simulink model "Microgrid_transition_model_111821_ben"  (R2020a)
settings: Solver=VariableStepAuto  StartTime=0.0  StopTime=16  MaxStep=1e-4  RelTol=1e-3
PreLoadFcn:
  | %run('FC_microgrid_param.m')
  | %load('gen_grid_init.mat')
InitFcn:
  | %load myisoModel_init;
  | run('FC_microgrid_param.m')
  | tic
  | run('CARTinitFcn.m')
  | %caseNo = 2;
  | 
  | %if (caseNo == 1)
  | %set_param(['Isolated_grid_paper_model_022521/SignalGen'], 'ActiveScenario', 'PStep222kW');
  | %else
  | %set_param(['Isolated_grid_paper_model_022521/SignalGen'], 'ActiveScenario', 'QStep222kVAr');
  | 
  | %end;
StopFcn:
  | toc
undefined symbols (not defined in the file): breakpoints1, breakpoints2, cc_kp, cp_table_data, ctrl, D1, Delta, DiscIntNeverNeededParam, DT, FC_BESS, FC_PV_FirstSolar, find_system, gcbh, libFC_BESS, libFC_PV, LowerLimit, magnitude, oversize, pll_ki, pll_kp, pq_ts, sps_rtmsupport, timer, Ts, ts, Ts_APC, Ts_Control, Ts_Power, UpperLimit
libraries: powerlib x152, powerlib_extras x100, simulink x95, powerlib_meascontrol x86, eePowerMeasurement x26, pi_ctrl x16, simulink_extras x12, sps_avr x7, spsDieselMotorModel x3, libFSArray x2, SignalEditorBlockLib x2, libLgBattery x1
(part 9 of 14)

== system Microgrid_transition_model_111821_ben/Wind Turbine Type 4/Control/Grid-Side Inverter Control/PI with anti-windup and dynamic limits - Iq ==
  note: Aramis Schwanka Trevisan - 16.08.2016
      | PI-controller with anti-windup and dynamic limits
      | Update 17.12.2016: External reset
      | Update 21.02.2017: External reset + limitation
  UpperLimit : Inport
  Input : Inport  Port=2
  LowerLimit : Inport  Port=3
  Reset : Inport  Port=4
  x_reset : Inport  Port=5
  Add1 : Sum
  Add2 : Sum
  Add3 : Sum  Inputs=+++
  Compare To Zero : simulink/Logic and Bit Operations/Compare To Zero  relop=>  OutDataTypeStr=uint8  ZeroCross=off
  Compare To Zero1 : simulink/Logic and Bit Operations/Compare To Zero  relop=<  OutDataTypeStr=uint8  ZeroCross=off
  Constant : Constant  Value=0
  Discrete Integrator : DiscreteIntegrator  IntegratorMethod=Integration: Trapezoidal  gainval=1  ExternalReset=sampled level  InitialConditionSource=external  InitialCondition=Init  SampleTime=Ts  UpperSaturationLimit=UpperLimit  LowerSaturationLimit=LowerLimit  ShowStatePort=on  ICPrevOutput=DiscIntNeverNeededParam  ICPrevScaledInput=DiscIntNeverNeededParam
  IC : InitialCondition  Value=Init
  Kp1 : Gain  Gain=Kp  SaturateOnIntegerOverflow=on  SampleTime=Ts  OutDataTypeStr=Inherit: Same as input  ParamDataTypeStr=Inherit: Same as input
  Kp5 : Gain  Gain=Ki  SaturateOnIntegerOverflow=on  SampleTime=Ts  OutDataTypeStr=Inherit: Same as input  ParamDataTypeStr=Inherit: Same as input
  Logical Operator : Logic  AllPortsSameDT=off  OutDataTypeStr=boolean
  Logical Operator1 : Logic  AllPortsSameDT=off  OutDataTypeStr=boolean
  Logical Operator2 : Logic  Operator=OR  AllPortsSameDT=off  OutDataTypeStr=boolean
  Logical Operator3 : Logic  Operator=OR  Inputs=3  AllPortsSameDT=off  OutDataTypeStr=boolean
  Logical Operator4 : Logic  Operator=NOT  Inputs=3  AllPortsSameDT=off  OutDataTypeStr=boolean
  Product : Product  Inputs=3
  Product1 : Product  Inputs=3
  Product2 : Product
  Relational Operator : RelationalOperator  OutDataTypeStr=boolean  RndMeth=Nearest
  Relational Operator1 : RelationalOperator  Operator=<=  OutDataTypeStr=boolean  RndMeth=Nearest
  Relational Operator2 : RelationalOperator  OutDataTypeStr=boolean  RndMeth=Nearest
  Relational Operator3 : RelationalOperator  Operator=<=  OutDataTypeStr=boolean  RndMeth=Nearest
  Saturation Dynamic : simulink/Discontinuities/Saturation Dynamic  OutMin=[]  OutMax=[]  OutDataTypeStr=Inherit: Same as second input  OutDataType=fixdt(1, 16)  OutScaling=2^-10  DoSatur=off
  Switch : Switch  Criteria=u2 > Threshold
  Zero-Order Hold : ZeroOrderHold  SampleTime=Ts
  Output : Outport
  wires:
  Saturation Dynamic/1 -> Output/1
  Reset/1 -> Product2/2, Logical Operator3/3, Logical Operator4/1
  IC/1 -> Discrete Integrator/3
  Switch/1 -> Discrete Integrator/1
  Compare To Zero1/1 -> Logical Operator1/2  "Error_is_negative"
  Logical Operator/1 -> Logical Operator2/1
  Relational Operator/1 -> Logical Operator/1  "UpperLimit_is_Reached"
  Relational Operator1/1 -> Logical Operator1/1  "LowerLimit_Is_Reached"
  Logical Operator2/1 -> Switch/2
  Kp1/1 -> Zero-Order Hold/1
  Constant/1 -> Switch/1
  Kp5/1 -> Switch/3
  Add2/1 -> Saturation Dynamic/2
  Zero-Order Hold/1 -> Add2/1, Add1/2
  Add1/1 -> Relational Operator/1, Relational Operator1/1
  Input/1 -> Kp5/1, Compare To Zero1/1, Compare To Zero/1, Kp1/1
  Compare To Zero/1 -> Logical Operator/2  "Error_is_positive"
  Logical Operator1/1 -> Logical Operator2/2
  Relational Operator2/1 -> Logical Operator3/1, Product/2
  Relational Operator3/1 -> Product1/2, Logical Operator3/2
  Logical Operator3/1 -> Discrete Integrator/2
  Add3/1 -> IC/1
  Product1/1 -> Add3/2
  UpperLimit/1 -> Saturation Dynamic/1, Relational Operator/2, Product/1, Relational Operator2/2
  Discrete Integrator/State -> Add1/1, Relational Operator3/1, Relational Operator2/1
  Discrete Integrator/1 -> Add2/2
  Logical Operator4/1 -> Product/3, Product1/1
  LowerLimit/1 -> Saturation Dynamic/3, Relational Operator1/2, Relational Operator3/2, Product1/3
  Product2/1 -> Add3/3
  Product/1 -> Add3/1
  x_reset/1 -> Product2/1

== system Microgrid_transition_model_111821_ben/Wind Turbine Type 4/Control/Grid-Side Inverter Control/Predictor1 ==
  in : Inport
  Delay : Delay  DelayLength=1  InitialCondition=Init_value  SampleTime=Ts
  Delay1 : Delay  DelayLength=1  InitialCondition=Init_value  SampleTime=Ts
  Gain : Gain  Gain=2
  Sum1 : Sum  Inputs=|+-
  out : Outport
  wires:
  in/1 -> Delay/1
  Delay1/1 -> Sum1/2
  Sum1/1 -> out/1
  Delay/1 -> Gain/1, Delay1/1
  Gain/1 -> Sum1/1

== system Microgrid_transition_model_111821_ben/Wind Turbine Type 4/Control/Grid-Side Inverter Control/Predictor2 ==
  in : Inport
  Delay : Delay  DelayLength=1  InitialCondition=Init_value  SampleTime=Ts
  Delay1 : Delay  DelayLength=1  InitialCondition=Init_value  SampleTime=Ts
  Gain : Gain  Gain=2
  Sum1 : Sum  Inputs=|+-
  out : Outport
  wires:
  Gain/1 -> Sum1/1
  Delay/1 -> Delay1/1, Gain/1
  Sum1/1 -> out/1
  Delay1/1 -> Sum1/2
  in/1 -> Delay/1

== system Microgrid_transition_model_111821_ben/Wind Turbine Type 4/Control/Measurement and Transformation/Discrete 3-phase PLL-Driven Positive-Sequence Active & Reactive Power ==
  note: Pierre Giroux, Gilbert Sybille
      | Power System Simulation Laboratory
      | IREQ, Hydro-Quebc
  note: Discrete 3-phase PLL-driven Positive-Sequence Active & Reactive Power
  Freq : Inport  PortDimensions=1
  w : Inport  Port=2  PortDimensions=1
  Vabc : Inport  Port=3  PortDimensions=3
  Iabc : Inport  Port=4  PortDimensions=3
  Deg->Rad : Gain  Gain=pi/180  SaturateOnIntegerOverflow=on  OutDataTypeStr=Inherit: Same as input  ParamDataTypeStr=Inherit: Same as input
  Discrete 3-phase PLL-Driven Positive-Sequence Fundamental Value : Subsystem  mask(Discrete 3-phase PLL-Driven Positive-Sequence Fundamental Value){Finit=Finit, Fmin=Fmin, Par_Init=Par_Vinit, Ts=Ts}
      mask prompts: Finit "Initial frequency (Hz):"; Fmin "Minimum frequency (Hz):"; Par_Init "Initial input (positive component): [ Mag  Phase-relative-to-PLL(degrees) ]"; Ts "Sample time:"
      mask help:
      | For a supplied fundamental frequency (port Freq), this discrete block computes  the positive-sequence component (Magnitude and Phase)  of a set of three balanced or unbalanced signals (port abc) which may contain harmonics.
      |  Input port "Sin_Cos" (a two-dimension signal) provides the reference frame required for the computation..
      |  First and second outputs return respectively the magnitude and phase (in degrees relative to the PLL phase)) of the fundamental.
      | For the first cycle of simulation, the outputs are held constant to the values specified by the parameter "Initial input".
      | constant to the values specified by the parameter "Initial input". The value of the parameter "Minimum frequency" is used to determine the buffer size of the "Variable Transport Delay" block found inside this subsystem.
      mask init:
      | Real_Init=Par_Init(1)*cos(pi/180*Par_Init(2));
      | Imag_Init=Par_Init(1)*sin(pi/180*Par_Init(2));
      | power_initmask();
      settings: OpenFcn=power_openblockproxy();
  Discrete 3-phase PLL-Driven Positive-Sequence Fundamental Value2 : Subsystem  mask(Discrete 3-phase PLL-Driven Positive-Sequence Fundamental Value){Finit=Finit, Fmin=Fmin, Par_Init=Par_Iinit, Ts=Ts}
      mask prompts: Finit "Initial frequency (Hz):"; Fmin "Minimum frequency (Hz):"; Par_Init "Initial input (positive component): [ Mag  Phase-relative-to-PLL(degrees) ]"; Ts "Sample time:"
      mask help:
      | For a supplied fundamental frequency (port Freq), this discrete block computes  the positive-sequence component (Magnitude and Phase)  of a set of three balanced or unbalanced signals (port abc) which may contain harmonics.
      |  Input port "Sin_Cos" (a two-dimension signal) provides the reference frame required for the computation..
      |  First and second outputs return respectively the magnitude and phase (in degrees relative to the PLL phase)) of the fundamental.
      | For the first cycle of simulation, the outputs are held constant to the values specified by the parameter "Initial input".
      | constant to the values specified by the parameter "Initial input". The value of the parameter "Minimum frequency" is used to determine the buffer size of the "Variable Transport Delay" block found inside this subsystem.
      mask init:
      | Real_Init=Par_Init(1)*cos(pi/180*Par_Init(2));
      | Imag_Init=Par_Init(1)*sin(pi/180*Par_Init(2));
      | power_initmask();
      settings: OpenFcn=power_openblockproxy();
  Gain1 : Gain  Gain=3/2  SaturateOnIntegerOverflow=on  OutDataTypeStr=Inherit: Same as input  ParamDataTypeStr=Inherit: Same as input
  Mux2 : Mux  Inputs=2
  Mux3 : Mux  Inputs=2
  Product : Product  InputSameDT=on  SaturateOnIntegerOverflow=on  OutDataTypeStr=Inherit: Same as first input
  Product1 : Product  InputSameDT=on  SaturateOnIntegerOverflow=on  OutDataTypeStr=Inherit: Same as first input
  Product2 : Product  InputSameDT=on  SaturateOnIntegerOverflow=on  OutDataTypeStr=Inherit: Same as first input
  Sum : Sum  Inputs=+-  InputSameDT=on  SaturateOnIntegerOverflow=on  OutDataTypeStr=Inherit: Same as first input
  Trigonometric Function : Trigonometry
  Trigonometric Function1 : Trigonometry  Operator=cos
  Mag_V_I : Outport  VectorParamsAs1DForOutWhenUnconnected=off
  P_Q : Outport  Port=2  VectorParamsAs1DForOutWhenUnconnected=off
  wires:
  Iabc/1 -> Discrete 3-phase PLL-Driven Positive-Sequence Fundamental Value2/3(abc)
  Discrete 3-phase PLL-Driven Positive-Sequence Fundamental Value2/1(Mag) -> Product2/2, Mux3/2
  Product2/1 -> Product1/2, Product/1
  Gain1/1 -> P_Q/1
  Mux3/1 -> Mag_V_I/1
  Product1/1 -> Mux2/2
  Product/1 -> Mux2/1
  Mux2/1 -> Gain1/1
  Trigonometric Function/1 -> Product1/1
  Trigonometric Function1/1 -> Product/2
  Deg->Rad/1 -> Trigonometric Function/1, Trigonometric Function1/1
  Sum/1 -> Deg->Rad/1
  Discrete 3-phase PLL-Driven Positive-Sequence Fundamental Value2/2(Phase) -> Sum/2
  Discrete 3-phase PLL-Driven Positive-Sequence Fundamental Value/1(Mag) -> Product2/1, Mux3/1
  Discrete 3-phase PLL-Driven Positive-Sequence Fundamental Value/2(Phase) -> Sum/1
  w/1 -> Discrete 3-phase PLL-Driven Positive-Sequence Fundamental Value2/2(w), Discrete 3-phase PLL-Driven Positive-Sequence Fundamental Value/2(w)
  Freq/1 -> Discrete 3-phase PLL-Driven Positive-Sequence Fundamental Value2/1(Freq), Discrete 3-phase PLL-Driven Positive-Sequence Fundamental Value/1(Freq)
  Vabc/1 -> Discrete 3-phase PLL-Driven Positive-Sequence Fundamental Value/3(abc)

== system Microgrid_transition_model_111821_ben/Wind Turbine Type 4/Control/Measurement and Transformation/Extract References ==
  v_abc : Inport
  Extract References : Subsystem
  Mux : Mux  Inputs=3
  Voltage and Frequency Protection : Subsystem
  rad/s to Hz : Gain  Gain=1/2/pi
  u_frt_pu : Outport
  protection_u_f : Outport  Port=2
  references : Outport  Port=3
  wires:
  Extract References/4(u_frt_pu) -> u_frt_pu/1
  Extract References/2(wt_ref) -> Mux/2
  Extract References/3(w_ref) -> rad/s to Hz/1, Mux/3
  Mux/1 -> references/1
  [Vpos] -> Voltage and Frequency Protection/1(Vpos)
  [fgrid] -> Voltage and Frequency Protection/2(fgrid)
  Voltage and Frequency Protection/1(u_f_protect) -> protection_u_f/1
  Extract References/1(u_ref) -> [Vpos], Mux/1
  rad/s to Hz/1 -> [fgrid]
  v_abc/1 -> Extract References/1(v_abc)

== system Microgrid_transition_model_111821_ben/Wind Turbine Type 4/Control/Measurement and Transformation/Filter ==
  Vabc_grid : Inport
  Iabc_grid_conv : Inport  Port=2
  Vabc_LL_s : Inport  Port=3
  Iabc_stator : Inport  Port=4
  IL : Inport  Port=5
  Vdc : Inport  Port=6
  Qref : Inport  Port=7
  wr : Inport  Port=8
  angle_rotor : Inport  Port=9
  Second-Order Filter{,1..6} (7 alike) : powerlib_meascontrol/Filters/Second-Order Filter  FilterType=Lowpass  Fo=Freq  Zeta=Zeta  Ts=Ts  Initialize=off  Vac_Init="[0,  0,  60]"  Vdc_Init=0  PlotResponse=off  FreqRange=[0, 500, 1]
      settings: SourceProductBaseCode=MT,PS
  Second-Order Filter7 : powerlib_meascontrol/Filters/Second-Order Filter  FilterType=Lowpass  Fo=Freq  Zeta=Zeta  Ts=Ts  Initialize=on  Vac_Init=[0.8 -25 60]*0  Vdc_Init=Vdc_nom  PlotResponse=off  FreqRange=[0, 500, 1]
      settings: SourceProductBaseCode=MT,PS
  Second-Order Filter8 : powerlib_meascontrol/Filters/Second-Order Filter  FilterType=Lowpass  Fo=Freq  Zeta=Zeta  Ts=Ts  Initialize=on  Vac_Init=[0.8 -25 60]*0  Vdc_Init=1+init(1)/100  PlotResponse=off  FreqRange=[0, 500, 1]
      settings: SourceProductBaseCode=MT,PS
  "Vabc_grid " : Outport  VectorParamsAs1DForOutWhenUnconnected=off
  "Iabc_grid_conv " : Outport  Port=2  VectorParamsAs1DForOutWhenUnconnected=off
  "Vabc_LL_s " : Outport  Port=3  VectorParamsAs1DForOutWhenUnconnected=off
  "Iabc_stator " : Outport  Port=4  VectorParamsAs1DForOutWhenUnconnected=off
  "IL " : Outport  Port=5  VectorParamsAs1DForOutWhenUnconnected=off
  "Vdc " : Outport  Port=6  VectorParamsAs1DForOutWhenUnconnected=off
  "Qref " : Outport  Port=7  VectorParamsAs1DForOutWhenUnconnected=off
  "wr " : Outport  Port=8  VectorParamsAs1DForOutWhenUnconnected=off
  "angle_rotor " : Outport  Port=9  VectorParamsAs1DForOutWhenUnconnected=off
  wires:
  angle_rotor/1 -> Second-Order Filter6/1
  Second-Order Filter6/1 -> "angle_rotor "/1
  Second-Order Filter/1 -> "Vabc_grid "/1
  Second-Order Filter1/1 -> "Iabc_grid_conv "/1
  Vdc/1 -> Second-Order Filter7/1
  Second-Order Filter7/1 -> "Vdc "/1
  Second-Order Filter3/1 -> "Iabc_stator "/1
  wr/1 -> Second-Order Filter8/1
  Second-Order Filter8/1 -> "wr "/1
  Qref/1 -> Second-Order Filter5/1
  Second-Order Filter5/1 -> "Qref "/1
  IL/1 -> Second-Order Filter4/1
  Second-Order Filter4/1 -> "IL "/1
  Vabc_grid/1 -> Second-Order Filter/1
  Iabc_grid_conv/1 -> Second-Order Filter1/1
  Vabc_LL_s/1 -> Second-Order Filter2/1
  Second-Order Filter2/1 -> "Vabc_LL_s "/1
  Iabc_stator/1 -> Second-Order Filter3/1

== system Microgrid_transition_model_111821_ben/Wind Turbine Type 4/Control/Measurement and Transformation/Stator flux estimator ==
  note: Quasi steady state flux at generator stator
  Vdqs : Inport
  Idqs : Inport  Port=2
  wr : Inport  Port=3
  Divide2 : Product  Inputs=**
  Divide4 : Product  Inputs=*/
  Divide7 : Product  Inputs=**
  Divide8 : Product  Inputs=*/
  First-Order Filter : powerlib_meascontrol/Filters/First-Order Filter  FilterType=Lowpass  Tc=Flux_meas_time_constant  Ts=Ts  Initialize=on  Vac_Init=[0, 0, 0]  Vdc_Init=1  PlotResponse=off  FreqRange="[0,  200,  1]"
      settings: SourceProductBaseCode=MT,PS
  Gain : Gain  Gain=-1
  Magnitude of flux : Fcn  Expr=sqrt(u(1)^2+u(2)^2)
  Mux1 : Mux  Inputs=2
  Rs2 : Constant  Value=Resistance
  Rs4 : Constant  Value=Resistance
  Selector1 : Selector  InputPortWidth=2  IndexOptions=Index vector (dialog)  Indices=2  OutputSizes=1
  Selector3 : Selector  InputPortWidth=2  IndexOptions=Index vector (dialog)  Indices=2  OutputSizes=1
  Selector7 : Selector  InputPortWidth=2  IndexOptions=Index vector (dialog)  Indices=1  OutputSizes=1
  Selector8 : Selector  InputPortWidth=2  IndexOptions=Index vector (dialog)  Indices=1  OutputSizes=1
  Sum2 : Sum  Inputs=|+-
  Sum4 : Sum  Inputs=|+-
  avoid division by 0 : Saturate  UpperLimit=inf  LowerLimit=1e-6
  Flux : Outport  VectorParamsAs1DForOutWhenUnconnected=off
  wires:
  First-Order Filter/1 -> Flux/1
  avoid division by 0/1 -> Gain/1, Divide4/2
  Magnitude of flux/1 -> First-Order Filter/1
  Mux1/1 -> Magnitude of flux/1
  Divide8/1 -> Mux1/2  "phi_q"
  Gain/1 -> Divide8/2
  Sum4/1 -> Divide8/1
  Selector8/1 -> Divide7/1  "Id"
  Rs4/1 -> Divide7/2
  Selector7/1 -> Sum4/1  "Vd"
  Divide7/1 -> Sum4/2  "Rs*Id"
  Idqs/1 -> Selector8/1, Selector3/1
  Vdqs/1 -> Selector7/1, Selector1/1
  Selector3/1 -> Divide2/1  "Iq"
  Rs2/1 -> Divide2/2
  Selector1/1 -> Sum2/1  "Vq"
  Divide2/1 -> Sum2/2  "Rs*Iq"
  Divide4/1 -> Mux1/1  "phi_d"
  Sum2/1 -> Divide4/1
  wr/1 -> avoid division by 0/1

== system Microgrid_transition_model_111821_ben/Wind Turbine Type 4/Control/Measurement and Transformation/abc2qd ==
  note: This subsystem converts Vab and Vbc to Vd,Vq. The sine and cosine com-
      | puted here are sent to the inverse transformation subsystem qd/abc.
  Vabc_LL : Inport
  sin_cos : Inport  Port=2
  Fcn2 : Fcn  Expr=(u[4]*(2*u[1]+u[2]) + (sqrt(3)*u[2]*u[3])) * 1/3
  Fcn3 : Fcn  Expr=(u[3]*(2*u[1]+u[2]) + (-sqrt(3)*u[2]*u[4])) * 1/3
  Mux : Mux  Inputs=2
  Mux1 : Mux  Inputs=[ 2 2 ]
  Selector : Selector  InputPortWidth=3  IndexOptions=Index vector (dialog)  Indices=[1 2]  OutputSizes=1
  Vdq : Outport  InitialOutput=0  VectorParamsAs1DForOutWhenUnconnected=off
  wires:
  Fcn3/1 -> Mux/1
  Fcn2/1 -> Mux/2
  Mux1/1 -> Fcn3/1, Fcn2/1
  Vabc_LL/1 -> Selector/1
  sin_cos/1 -> Mux1/2
  Mux/1 -> Vdq/1
  Selector/1 -> Mux1/1

== system Microgrid_transition_model_111821_ben/Wind Turbine Type 4/Control/Speed & Pitch Control1/Discrete PI Controller1 ==
  note: Discrete PID Controller
  note: Pierre Giroux, Gilbert Sybille
      | Power System Simulation Laboratory
      | IREQ, Hydro-Quebc
  Error : Inport  SampleTime=Ts
  Discrete-Time Integrator : DiscreteIntegrator  InitialCondition=Init  SampleTime=Ts  LimitOutput=on  UpperSaturationLimit=UpperLimit  LowerSaturationLimit=LowerLimit  ICPrevOutput=DiscIntNeverNeededParam  ICPrevScaledInput=DiscIntNeverNeededParam
  Kp4 : Gain  Gain=Kp  SaturateOnIntegerOverflow=on  SampleTime=Ts  OutDataTypeStr=Inherit: Same as input  ParamDataTypeStr=Inherit: Same as input
  Kp5 : Gain  Gain=Ki  SaturateOnIntegerOverflow=on  SampleTime=Ts  OutDataTypeStr=Inherit: Same as input  ParamDataTypeStr=Inherit: Same as input
  Saturation2 : Saturate  UpperLimit=UpperLimit  LowerLimit=LowerLimit  SampleTime=Ts
  Sum6 : Sum  InputSameDT=on  SaturateOnIntegerOverflow=on  SampleTime=Ts  OutDataTypeStr=Inherit: Same as first input
  Zero-Order Hold : ZeroOrderHold  SampleTime=Ts
  Out : Outport  SampleTime=Ts  InitialOutput=0  VectorParamsAs1DForOutWhenUnconnected=off
  wires:
  Zero-Order Hold/1 -> Sum6/1
  Saturation2/1 -> Out/1
  Discrete-Time Integrator/1 -> Sum6/2
  Kp4/1 -> Zero-Order Hold/1
  Kp5/1 -> Discrete-Time Integrator/1
  Sum6/1 -> Saturation2/1
  Error/1 -> Kp5/1, Kp4/1

== system Microgrid_transition_model_111821_ben/Wind Turbine Type 4/Control/Speed & Pitch Control1/Discrete PI Controller2 ==
  note: Discrete PID Controller
  note: Pierre Giroux, Gilbert Sybille
      | Power System Simulation Laboratory
      | IREQ, Hydro-Quebc
  Error : Inport  SampleTime=Ts
  Discrete-Time Integrator : DiscreteIntegrator  InitialCondition=Init  SampleTime=Ts  LimitOutput=on  UpperSaturationLimit=UpperLimit  LowerSaturationLimit=LowerLimit  ICPrevOutput=DiscIntNeverNeededParam  ICPrevScaledInput=DiscIntNeverNeededParam
  Kp4 : Gain  Gain=Kp  SaturateOnIntegerOverflow=on  SampleTime=Ts  OutDataTypeStr=Inherit: Same as input  ParamDataTypeStr=Inherit: Same as input
  Kp5 : Gain  Gain=Ki  SaturateOnIntegerOverflow=on  SampleTime=Ts  OutDataTypeStr=Inherit: Same as input  ParamDataTypeStr=Inherit: Same as input
  Saturation2 : Saturate  UpperLimit=UpperLimit  LowerLimit=LowerLimit  SampleTime=Ts
  Sum6 : Sum  InputSameDT=on  SaturateOnIntegerOverflow=on  SampleTime=Ts  OutDataTypeStr=Inherit: Same as first input
  Zero-Order Hold : ZeroOrderHold  SampleTime=Ts
  Out : Outport  SampleTime=Ts  InitialOutput=0  VectorParamsAs1DForOutWhenUnconnected=off
  wires:
  Zero-Order Hold/1 -> Sum6/1
  Saturation2/1 -> Out/1
  Discrete-Time Integrator/1 -> Sum6/2
  Kp4/1 -> Zero-Order Hold/1
  Kp5/1 -> Discrete-Time Integrator/1
  Sum6/1 -> Saturation2/1
  Error/1 -> Kp5/1, Kp4/1

== system Microgrid_transition_model_111821_ben/../Control/Grid-side converter Control system/INT/S6 ==
  note: Limiter
      | with external
      | limits
  MAX : Inport
  In : Inport  Port=2
  MIN : Inport  Port=3
  MinMax : MinMax  Function=max  Inputs=2  InputSameDT=on  SaturateOnIntegerOverflow=on
  MinMax1 : MinMax  Inputs=2  InputSameDT=on  SaturateOnIntegerOverflow=on
  "  " : Outport  InitialOutput=0  VectorParamsAs1DForOutWhenUnconnected=off
  wires:
  In/1 -> MinMax1/2
  MinMax/1 -> "  "/1
  MIN/1 -> MinMax/1
  MAX/1 -> MinMax1/1
  MinMax1/1 -> MinMax/2

== system Microgrid_transition_model_111821_ben/../Control/Measurement and Transformation/Discrete 3-phase PLL-Driven Positive-Sequence Active & Reactive Power/Discrete 3-phase PLL-Driven Positive-Sequence Fundamental Value ==
  note: Discrete 3-phase PLL-Driven Positive-Sequence Fundamental Value
  note: Pierre Giroux, Gilbert Sybille
      | Power System Simulation Laboratory
      | IREQ, Hydro-Quebc
  Freq : Inport
  w : Inport  Port=2  PortDimensions=1
  abc : Inport  Port=3  PortDimensions=3
  Cartesian to Polar : simulink_extras/Transformations/Cartesian to Polar
  Demux : Demux  Outputs=3
      settings: DisplayOption=none
  Discrete Variable Frequency Mean value1 : Subsystem  mask(Discrete Variable-Frequency Mean Value){Finit=Finit, Fmin=Fmin, Vinit=Imag_Init, Ts=Ts}
      mask prompts: Finit "Initial frequency (Hz):"; Fmin "Minimum frequency (Hz):"; Vinit "Initial input (DC component):"; Ts "Sample time:"
      mask help:
      | This discrete block computes the mean value of the input signal (port In) over a running window of one cycle of a specified frequency (port Freq).
      |
      | For the first cycle of simulation (specified by the parameter "Initial frequency"), the output is held to the value of the  "Initial input" parameter.
      |
      | The value of the parameter "Minimum frequency" is used to determine the buffer size of the "Variable Transport Delay" block found inside this subsystem.
      mask init:
      | MaxDelay=1/Fmin+Ts;
      | power_initmask();
      settings: OpenFcn=power_openblockproxy();
  Discrete Variable Frequency Mean value2 : Subsystem  mask(Discrete Variable-Frequency Mean Value){Finit=Finit, Fmin=Fmin, Vinit=Real_Init, Ts=Ts}
      mask prompts: Finit "Initial frequency (Hz):"; Fmin "Minimum frequency (Hz):"; Vinit "Initial input (DC component):"; Ts "Sample time:"
      mask help:
      | This discrete block computes the mean value of the input signal (port In) over a running window of one cycle of a specified frequency (port Freq).
      |
      | For the first cycle of simulation (specified by the parameter "Initial frequency"), the output is held to the value of the  "Initial input" parameter.
      |
      | The value of the parameter "Minimum frequency" is used to determine the buffer size of the "Variable Transport Delay" block found inside this subsystem.
      mask init:
      | MaxDelay=1/Fmin+Ts;
      | power_initmask();
      settings: OpenFcn=power_openblockproxy();
  Rad->Deg. : Gain  Gain=180/pi  SaturateOnIntegerOverflow=on  OutDataTypeStr=Inherit: Same as input  ParamDataTypeStr=Inherit: Same as input
  Terminator : Terminator
  abc to dq0 : powerlib_meascontrol/Transformations/abc to dq0  Alignment=90 degrees behind phase A axis
      settings: SourceProductBaseCode=MT,PS
  Mag : Outport  VectorParamsAs1DForOutWhenUnconnected=off
  Phase : Outport  Port=2  VectorParamsAs1DForOutWhenUnconnected=off
  wires:
  Cartesian to Polar/2 -> Rad->Deg./1
  Cartesian to Polar/1 -> Mag/1
  Demux/3 -> Terminator/1
  abc to dq0/1 -> Demux/1
  abc/1 -> abc to dq0/1
  Demux/1 -> Discrete Variable Frequency Mean value2/2(In)
  Demux/2 -> Discrete Variable Frequency Mean value1/2(In)
  Discrete Variable Frequency Mean value1/1(Mean) -> Cartesian to Polar/2  "Real"
  Rad->Deg./1 -> Phase/1
  Discrete Variable Frequency Mean value2/1(Mean) -> Cartesian to Polar/1  "Real"
  Freq/1 -> Discrete Variable Frequency Mean value1/1(Freq), Discrete Variable Frequency Mean value2/1(Freq)
  w/1 -> abc to dq0/2

== system Microgrid_transition_model_111821_ben/../Control/Measurement and Transformation/Discrete 3-phase PLL-Driven Positive-Sequence Active & Reactive Power/Discrete 3-phase PLL-Driven Positive-Sequence Fundamental Value2 ==
  note: Pierre Giroux, Gilbert Sybille
      | Power System Simulation Laboratory
      | IREQ, Hydro-Quebc
  note: Discrete 3-phase PLL-Driven Positive-Sequence Fundamental Value
  Freq : Inport
  w : Inport  Port=2  PortDimensions=1
  abc : Inport  Port=3  PortDimensions=3
  Cartesian to Polar : simulink_extras/Transformations/Cartesian to Polar
  Demux : Demux  Outputs=3
      settings: DisplayOption=none
  Discrete Variable Frequency Mean value1 : Subsystem  mask(Discrete Variable-Frequency Mean Value){Finit=Finit, Fmin=Fmin, Vinit=Imag_Init, Ts=Ts}
      mask prompts: Finit "Initial frequency (Hz):"; Fmin "Minimum frequency (Hz):"; Vinit "Initial input (DC component):"; Ts "Sample time:"
      mask help:
      | This discrete block computes the mean value of the input signal (port In) over a running window of one cycle of a specified frequency (port Freq).
      |
      | For the first cycle of simulation (specified by the parameter "Initial frequency"), the output is held to the value of the  "Initial input" parameter.
      |
      | The value of the parameter "Minimum frequency" is used to determine the buffer size of the "Variable Transport Delay" block found inside this subsystem.
      mask init:
      | MaxDelay=1/Fmin+Ts;
      | power_initmask();
      settings: OpenFcn=power_openblockproxy();
  Discrete Variable Frequency Mean value2 : Subsystem  mask(Discrete Variable-Frequency Mean Value){Finit=Finit, Fmin=Fmin, Vinit=Real_Init, Ts=Ts}
      mask prompts: Finit "Initial frequency (Hz):"; Fmin "Minimum frequency (Hz):"; Vinit "Initial input (DC component):"; Ts "Sample time:"
      mask help:
      | This discrete block computes the mean value of the input signal (port In) over a running window of one cycle of a specified frequency (port Freq).
      |
      | For the first cycle of simulation (specified by the parameter "Initial frequency"), the output is held to the value of the  "Initial input" parameter.
      |
      | The value of the parameter "Minimum frequency" is used to determine the buffer size of the "Variable Transport Delay" block found inside this subsystem.
      mask init:
      | MaxDelay=1/Fmin+Ts;
      | power_initmask();
      settings: OpenFcn=power_openblockproxy();
  Rad->Deg. : Gain  Gain=180/pi  SaturateOnIntegerOverflow=on  OutDataTypeStr=Inherit: Same as input  ParamDataTypeStr=Inherit: Same as input
  Terminator : Terminator
  abc to dq0 : powerlib_meascontrol/Transformations/abc to dq0  Alignment=90 degrees behind phase A axis
      settings: SourceProductBaseCode=MT,PS
  Mag : Outport  VectorParamsAs1DForOutWhenUnconnected=off
  Phase : Outport  Port=2  VectorParamsAs1DForOutWhenUnconnected=off
  wires:
  w/1 -> abc to dq0/2
  Freq/1 -> Discrete Variable Frequency Mean value2/1(Freq), Discrete Variable Frequency Mean value1/1(Freq)
  Discrete Variable Frequency Mean value2/1(Mean) -> Cartesian to Polar/1  "Real"
  Rad->Deg./1 -> Phase/1
  Discrete Variable Frequency Mean value1/1(Mean) -> Cartesian to Polar/2  "Real"
  Demux/2 -> Discrete Variable Frequency Mean value1/2(In)
  Demux/1 -> Discrete Variable Frequency Mean value2/2(In)
  abc/1 -> abc to dq0/1
  abc to dq0/1 -> Demux/1
  Demux/3 -> Terminator/1
  Cartesian to Polar/1 -> Mag/1
  Cartesian to Polar/2 -> Rad->Deg./1

== system Microgrid_transition_model_111821_ben/FC_BESS/SMAInverter/85_SMAControl/InvControl/40_V_Control ==
  Add1 : Sum  Inputs=+-
  Bus Creator : BusCreator  Inputs=1
  Bus Selector1 : BusSelector  OutputSignals=vdq0_inv  OutputAsBus=on
  Bus Selector8 : BusSelector  OutputSignals=use_csi,vdq
  Constant1 : Constant  Value=double(0)
  Constant2 : Constant  Value=10  OutDataTypeStr=double
  Demux : Demux  Outputs=2
  Demux1 : Demux  Outputs=2
  Logical Operator : Logic  Operator=NOT  Inputs=1  AllPortsSameDT=off  OutDataTypeStr=boolean
  Manual Switch2 : ManualSwitch  CurrentSetting=0
  Mux2 : Mux  Inputs=2
  Mux8 : Mux  Inputs=2
  PI_controller_with_reset : pi_ctrl/PI_controller_with_reset  Kp=0.0005  Ti=0.02  Ts=Ts  Iup=1.5  Idown=0  PIup=1.5  PIdown=0
  PI_controller_with_reset1 : pi_ctrl/PI_controller_with_reset  Kp=0.0005  Ti=0.02  Ts=Ts  Iup=1.5  Idown=-1  PIup=1.5  PIdown=-1
  Scope : Scope  NumInputPorts=4
  Selector : Selector  InputPortWidth=4  IndexOptions=Index vector (dialog)  Indices=2  OutputSizes=1
  Selector2 : Selector  InputPortWidth=3  IndexOptions=Index vector (dialog)  Indices=[1 2]  OutputSizes=1
  Subsystem : Subsystem  mask{Ts=Ts}
      mask prompts: Ts "Sampling time"
  Unit Delay : UnitDelay  SampleTime=-1  HasFrameUpgradeWarning=on
  Unit Delay1 : UnitDelay  InitialCondition=[0 0]  SampleTime=-1  HasFrameUpgradeWarning=on
  tag scope: V_Ctrl=scoped
  wires:
  Unit Delay1/1 -> Demux/1, Subsystem/3(init)
  Constant2/1 -> Subsystem/4(rate)
  Mux2/1 -> Subsystem/1(in)
  Bus Selector8/1 -> Logical Operator/1, Subsystem/2(rst)  "<use_csi>"
  Unit Delay/1 -> Manual Switch2/1
  Selector2/1 -> Manual Switch2/2
  Demux/2 -> PI_controller_with_reset1/3
  Demux/1 -> PI_controller_with_reset/3
  Bus Selector8/2 -> Unit Delay1/1  "<vdq>"
  Logical Operator/1 -> PI_controller_with_reset/2, PI_controller_with_reset1/2
  PI_controller_with_reset1/1 -> Mux8/2
  [inverter] -> Bus Selector8/1
  Constant1/1 -> Mux2/2
  Selector/1 -> Mux2/1
  Manual Switch2/1 -> Scope/2, Add1/2
  Subsystem/1(out) -> Scope/1, Add1/1
  Add1/1 -> Demux1/1
  Demux1/2 -> PI_controller_with_reset1/1
  Demux1/1 -> PI_controller_with_reset/1
  PI_controller_with_reset/1 -> Scope/4, Mux8/1
  Bus Selector1/1 -> Selector2/1
  [cb_meas] -> Bus Selector1/1
  Mux8/1 -> Bus Creator/1, Unit Delay/1, Scope/3  "udq"
  Bus Creator/1 -> [V_Ctrl]
  [ref_lim] -> Selector/1

== system Microgrid_transition_model_111821_ben/FC_BESS/SMAInverter/85_SMAControl/InvControl/50_I_Control ==
  Add1 : Sum  Inputs=+-
  Bus Creator : BusCreator  Inputs=1
  Bus Selector1 : BusSelector  OutputSignals=idq0  OutputAsBus=on
  Bus Selector2 : BusSelector  OutputSignals=use_csi,vdq
  Bus Selector3 : BusSelector  OutputSignals=vdq0  OutputAsBus=on
  Constant : Constant  Value=10  OutDataTypeStr=double
  Demux : Demux  Outputs=2
  Demux1 : Demux  Outputs=2
  Filter : Subsystem
  Filter1 : Subsystem
  Gain : Gain  Gain=0
  Gain1 : Gain  Gain=0
  Logical Operator : Logic  Operator=NOT  Inputs=1  AllPortsSameDT=off  OutDataTypeStr=boolean
  Mux8 : Mux  Inputs=2
  PI_controller_with_reset : pi_ctrl/PI_controller_with_reset  Kp=cc_kp  Ti=cc_Ti  Ts=Ts  Iup=1.5  Idown=-0.5  PIup=1.5  PIdown=-0.5
  PI_controller_with_reset1 : pi_ctrl/PI_controller_with_reset  Kp=cc_kp  Ti=0.6e-3*100  Ts=Ts  Iup=1  Idown=-1  PIup=1  PIdown=-1
  Scope : Scope  NumInputPorts=3
  Selector : Selector  InputPortWidth=4  IndexOptions=Index vector (dialog)  Indices=[3 4]  OutputSizes=1
  Selector1 : Selector  InputPortWidth=3  IndexOptions=Index vector (dialog)  Indices=[1 2]  OutputSizes=1
  Selector2 : Selector  InputPortWidth=3  IndexOptions=Index vector (dialog)  Indices=[1 2]  OutputSizes=1
  Subsystem : Subsystem  mask{Ts=Ts}
      mask prompts: Ts "Sampling time"
  Sum : Sum  Inputs=|++
  Sum1 : Sum  Inputs=|+-
  Unit Delay : UnitDelay  SampleTime=-1  HasFrameUpgradeWarning=on
  tag scope: I_Ctrl=scoped
  wires:
  PI_controller_with_reset1/1 -> Mux8/2
  Unit Delay/1 -> Sum1/1
  Logical Operator/1 -> Subsystem/2(rst)
  Constant/1 -> Subsystem/4(rate)
  Selector/1 -> Subsystem/1(in)
  Demux/2 -> PI_controller_with_reset1/3
  Demux/1 -> PI_controller_with_reset/3
  Bus Selector2/2 -> Unit Delay/1  "<vdq>"
  Bus Selector2/1 -> Logical Operator/1, PI_controller_with_reset1/2, Scope/1, PI_controller_with_reset/2  "<use_csi>"
  [inverter] -> Bus Selector2/1
  [ref_lim] -> Selector/1
  Bus Creator/1 -> [I_Ctrl]
  Sum/1 -> Scope/3, Bus Creator/1  "udq"
  [cb_meas] -> Bus Selector1/1
  Bus Selector1/1 -> Selector2/1
  PI_controller_with_reset/1 -> Mux8/1
  Demux1/1 -> PI_controller_with_reset/1
  Demux1/2 -> PI_controller_with_reset1/1
  Add1/1 -> Demux1/1
  Subsystem/1(out) -> Add1/1
  Selector2/1 -> Subsystem/3(init), Filter/1(In1)
  Filter/1(Out1) -> Add1/2
  Mux8/1 -> Sum/1, Scope/2  "udq"
  Sum1/1 -> Demux/1  "udq"
  [cb_meas] -> Bus Selector3/1
  Bus Selector3/1 -> Selector1/1
  Selector1/1 -> Filter1/1(In1)
  Filter1/1(Out1) -> Gain1/1, Gain/1
  Gain/1 -> Sum1/2
  Gain1/1 -> Sum/2

== system Microgrid_transition_model_111821_ben/FC_BESS/SMAInverter/85_SMAControl/InvControl/CB_Meas2 ==
  Bus Creator : BusCreator  Inputs=9
  Bus Selector1 : BusSelector  OutputSignals=vabc_line,iabc
  Bus Selector2 : BusSelector  OutputSignals=vabc_line
  Bus Selector3 : BusSelector  OutputSignals=ejwt
  Bus Selector4 : BusSelector  OutputSignals=iabc
  Bus Selector5 : BusSelector  OutputSignals=ejwt
  Bus Selector6 : BusSelector  OutputSignals=vabc_inv
  Bus Selector7 : BusSelector  OutputSignals=ejwt
  Filter : Subsystem
  Filter1 : Subsystem
  InvMeas : Scope  NumInputPorts=7
  Math Function : Math  Operator=square  SignedPower=on  SaturateOnIntegerOverflow=on
  Math Function1 : Math  Operator=square  SignedPower=on  SaturateOnIntegerOverflow=on
  PQ_Calculator : Subsystem
  Sqrt : Sqrt  SaturateOnIntegerOverflow=on
  Sqrt1 : Sqrt  SaturateOnIntegerOverflow=on
  Sum of Elements : Sum  Inputs=+
  Sum of Elements1 : Sum  Inputs=+
  Unit Delay : UnitDelay  SampleTime=-1  HasFrameUpgradeWarning=on
  Unit Delay1 : UnitDelay  SampleTime=-1  HasFrameUpgradeWarning=on
  Unit Delay2 : UnitDelay  SampleTime=-1  HasFrameUpgradeWarning=on
  abc_to_dq0 Transformation : powerlib_extras/Measurements/abc_to_dq0 Transformation
      settings: SourceProductBaseCode=PS
  abc_to_dq0 Transformation1 : powerlib_extras/Measurements/abc_to_dq0 Transformation
      settings: SourceProductBaseCode=PS
  abc_to_dq0 Transformation2 : powerlib_extras/Measurements/abc_to_dq0 Transformation
      settings: SourceProductBaseCode=PS
  tag scope: cb_meas=scoped
  wires:
  PQ_Calculator/2(Q - kVAR) -> Bus Creator/2, InvMeas/6  "q"
  Filter/1(Out1) -> Bus Creator/4, InvMeas/2, Math Function/1
  Filter1/1(Out1) -> Bus Creator/7, InvMeas/4, Math Function1/1
  abc_to_dq0 Transformation1/1 -> Bus Creator/6, InvMeas/3, Filter1/1(In1)  "idq0"
  abc_to_dq0 Transformation/1 -> Bus Creator/3, InvMeas/1, Filter/1(In1)  "vdq0"
  PQ_Calculator/1(P - kW) -> InvMeas/5, Bus Creator/1  "p"
  Unit Delay1/1 -> abc_to_dq0 Transformation1/2
  Unit Delay/1 -> abc_to_dq0 Transformation/2
  [cb_pu] -> Bus Selector4/1
  Sqrt1/1 -> Bus Creator/8  "irms"
  Sum of Elements1/1 -> Sqrt1/1
  Math Function1/1 -> Sum of Elements1/1
  Bus Selector5/1 -> Unit Delay1/1  "<ejwt>"
  [pll] -> Bus Selector5/1
  Bus Selector4/1 -> abc_to_dq0 Transformation1/1  "<iabc>"
  [cb_pu] -> Bus Selector2/1
  Sqrt/1 -> Bus Creator/5  "vrms"
  Sum of Elements/1 -> Sqrt/1
  Math Function/1 -> Sum of Elements/1
  Bus Selector3/1 -> Unit Delay/1  "<ejwt>"
  [pll] -> Bus Selector3/1
  Bus Selector2/1 -> abc_to_dq0 Transformation/1  "<vabc_line>"
  Bus Selector1/2 -> PQ_Calculator/2(Iabc)  "<iabc>"
  Bus Creator/1 -> [cb_meas]
  Bus Selector1/1 -> PQ_Calculator/1(Vabc)  "<vabc_line>"
  [cb_pu] -> Bus Selector1/1
  Bus Selector7/1 -> Unit Delay2/1  "<ejwt>"
  [pll] -> Bus Selector7/1
  [cb_pu] -> Bus Selector6/1
  Bus Selector6/1 -> abc_to_dq0 Transformation2/1  "<vabc_inv>"
  Unit Delay2/1 -> abc_to_dq0 Transformation2/2
  abc_to_dq0 Transformation2/1 -> InvMeas/7, Bus Creator/9  "vdq0_inv"

== system Microgrid_transition_model_111821_ben/FC_BESS/SMAInverter/85_SMAControl/InvControl/CB_pu ==
  Bus Creator : BusCreator  Inputs=3
  Bus Selector1 : BusSelector  OutputSignals=Uabc,Uabc_inv
  Bus Selector2 : BusSelector  OutputSignals=Iabc
  Gain : Gain  Gain=1/Unom/sqrt(2)
  Gain1 : Gain  Gain=1/Inom/sqrt(2)
  Gain2 : Gain  Gain=1/Unom/sqrt(2)
  tag scope: cb_pu=scoped
  wires:
  Gain1/1 -> Bus Creator/3  "iabc"
  Bus Selector2/1 -> Gain1/1  "<Iabc>"
  [inputs] -> Bus Selector2/1
  [inputs] -> Bus Selector1/1
  Bus Selector1/1 -> Gain/1  "<Uabc>"
  Gain/1 -> Bus Creator/1  "vabc_line"
  Bus Creator/1 -> [cb_pu]
  Bus Selector1/2 -> Gain2/1  "<Uabc_inv>"
  Gain2/1 -> Bus Creator/2  "vabc_inv"

== system Microgrid_transition_model_111821_ben/FC_BESS/SMAInverter/85_SMAControl/InvControl/CS_controller ==
  Bias : Bias  Bias=(1.5*Ts)*60*2*pi
  Bus Creator : BusCreator  Inputs=3
  Bus Selector10 : BusSelector  OutputSignals=cb_status,Control_Word.GF_mode
  Bus Selector2 : BusSelector  OutputSignals=udq
  Bus Selector3 : BusSelector  OutputSignals=udq
  Bus Selector5 : BusSelector  OutputSignals=wt
  Constant : Constant  Value=0
  Constant2 : Constant  Value=1.3
  Gain1 : Gain  Gain=-1
  Gain2 : Gain  Gain=Unom*sqrt(2)
  Logical Operator : Logic  AllPortsSameDT=off  OutDataTypeStr=boolean
  Logical Operator1 : Logic  Operator=NOT  AllPortsSameDT=off  OutDataTypeStr=boolean
  Mux1 : Mux  Inputs=2
  Mux3 : Mux  Inputs=2
  Saturation Dynamic : simulink/Discontinuities/Saturation Dynamic  OutMin=[]  OutMax=[]  OutDataTypeStr=Inherit: Same as second input  OutDataType=fixdt(1, 16)  OutScaling=2^-10  DoSatur=off
  Scope : Scope  NumInputPorts=2
  Switch : Switch  Criteria=u2 > Threshold
  Trigonometric Function2 : Trigonometry
  Trigonometric Function3 : Trigonometry  Operator=cos
  dq0_to_abc Transformation : powerlib_extras/Measurements/dq0_to_abc Transformation
      settings: SourceProductBaseCode=PS
  tag scope: inverter=scoped
  wires:
  [use_csi] -> Bus Creator/2  "use_csi"
  Bus Selector3/1 -> Switch/1  "<udq>"
  [I_Ctrl] -> Bus Selector3/1
  Logical Operator/1 -> Switch/2, Scope/1, [use_csi]
  [V_Ctrl] -> Bus Selector2/1
  Bus Selector2/1 -> Switch/3  "<udq>"
  [inputs] -> Bus Selector10/1
  Bus Selector10/2 -> Logical Operator1/1  "<GF_mode>"
  Logical Operator1/1 -> Logical Operator/2
  Bus Selector10/1 -> Logical Operator/1  "<cb_status>"
  Switch/1 -> Mux1/1, Bus Creator/3, Scope/2  "vdq"
  Mux1/1 -> dq0_to_abc Transformation/1
  Constant/1 -> Mux1/2
  Mux3/1 -> [ejwt]
  Trigonometric Function2/1 -> Mux3/1
  Trigonometric Function3/1 -> Mux3/2
  Bias/1 -> Trigonometric Function3/1, Trigonometric Function2/1
  Gain2/1 -> Bus Creator/1  "Uabc_ref"
  Constant2/1 -> Saturation Dynamic/1, Gain1/1
  Gain1/1 -> Saturation Dynamic/3
  Bus Creator/1 -> [inverter]
  dq0_to_abc Transformation/1 -> Saturation Dynamic/2
  [ejwt] -> dq0_to_abc Transformation/2
  Saturation Dynamic/1 -> Gain2/1  "uabc_ref"
  [pll] -> Bus Selector5/1
  Bus Selector5/1 -> Bias/1  "<wt>"

== system Microgrid_transition_model_111821_ben/FC_BESS/SMAInverter/85_SMAControl/InvControl/Droop ==
  Bus Selector1 : BusSelector  OutputSignals=vrms
  Bus Selector2 : BusSelector  OutputSignals=freq
  Bus Selector3 : BusSelector  OutputSignals=p,q,idq0
  Bus Selector9 : BusSelector  OutputSignals=fref,vref,pref,qref  OutputAsBus=on
  Constant : Constant  Value=[0 0]
  Demux : Demux
  Demux1 : Demux
  Droop : Subsystem
  ExtractCoefs : Subsystem
  Gain : Gain  Gain=[1 -1]
  Mux : Mux  Inputs=3
  Mux1 : Mux  Inputs=2
  Mux2 : Mux  Inputs=2
  Scope : Scope  NumInputPorts=4
  Scope1 : Scope  NumInputPorts=4
  Selector1 : Selector  InputPortWidth=4  IndexOptions=Index vector (dialog)  Indices=[1 2]  OutputSizes=1
  Selector2 : Selector  InputPortWidth=3  IndexOptions=Index vector (dialog)  Indices=[1 2]  OutputSizes=1
  Sum1 : Sum  Inputs=-+|
  Sum2 : Sum  Inputs=++|
  Terminator : Terminator
  tag scope: droop=scoped
  wires:
  Demux1/4 -> Scope1/4
  Demux1/1 -> Scope1/1
  Demux1/2 -> Scope1/2
  Demux1/3 -> Scope1/3
  Sum2/1 -> [droop], Demux1/1  "fvpq_meas"
  Gain/1 -> Mux/3
  Selector2/1 -> Gain/1
  Mux2/1 -> Terminator/1
  Bus Selector3/3 -> Selector2/1  "<idq0>"
  Bus Selector3/2 -> Mux2/2  "<q>"
  Bus Selector3/1 -> Mux2/1  "<p>"
  [cb_meas] -> Bus Selector3/1
  Demux/4 -> Scope/4
  Demux/3 -> Scope/3
  Demux/2 -> Scope/2
  Demux/1 -> Scope/1
  Bus Selector2/1 -> Mux/1  "<freq>"
  Bus Selector1/1 -> Mux/2  "<vrms>"
  [pll] -> Bus Selector2/1
  ExtractCoefs/1(Out1) -> Droop/2(droop)
  [inputs] -> ExtractCoefs/1(In1)
  Mux/1 -> Demux/1, Sum1/1  "fvpq_meas"
  [cb_meas] -> Bus Selector1/1
  Bus Selector9/1 -> Selector1/1, Sum2/2
  [inputs] -> Bus Selector9/1
  Droop/1(dFvpq_out) -> Sum2/1
  Sum1/1 -> Droop/1(dfvpq)
  Selector1/1 -> Mux1/1
  Mux1/1 -> Sum1/2
  Constant/1 -> Mux1/2

== system Microgrid_transition_model_111821_ben/FC_BESS/SMAInverter/85_SMAControl/InvControl/PLL ==
  note: Rising and falling edge debounce
  Aligned : simulink/Logic and Bit Operations/Interval Test  IntervalClosedRight=on  uplimit=0.05  IntervalClosedLeft=on  lowlimit=-0.05  OutDataTypeStr=boolean
  Aligned1 : simulink/Logic and Bit Operations/Interval Test  IntervalClosedRight=on  uplimit=1.25  IntervalClosedLeft=on  lowlimit=0.05  OutDataTypeStr=boolean
  Bus Creator : BusCreator  Inputs=5
  Bus Selector10 : BusSelector  OutputSignals=Control_Word.GF_mode
  Bus Selector2 : BusSelector  OutputSignals=vabc_line
  Bus Selector8 : BusSelector  OutputSignals=cb_status
  Constant : Constant  Value=0
  Data Type Conversion : DataTypeConversion
  DebounceAlternative : Subsystem  mask{Tdb_off=0.05, Tdb_on=0.2, Tdb_sample=Ts}
      mask prompts: Tdb_off "Debounce Time When OFF"; Tdb_on "Debounce Time When On"; Tdb_sample "Sample Time"
      mask Display: disp(['Debouncing unit\nTdb when off is ' num2str(Tdb_off) '\nTdb when on is ' num2str(Tdb_on)]);
  Display : Display
  Gain : Gain  Gain=1/60
  Gain1 : Gain  Gain=2*pi*60  SaturateOnIntegerOverflow=on  OutDataTypeStr=Inherit: Same as input  ParamDataTypeStr=Inherit: Same as input
  Logical Operator1 : Logic  AllPortsSameDT=off  OutDataTypeStr=boolean
  Logical Operator2 : Logic  AllPortsSameDT=off  OutDataTypeStr=boolean
  Logical Operator3 : Logic  AllPortsSameDT=off  OutDataTypeStr=boolean
  Logical Operator{4..6,8} (4 alike) : Logic  Operator=NOT  AllPortsSameDT=off  OutDataTypeStr=boolean
  Logical Operator7 : Logic  Operator=OR  AllPortsSameDT=off  OutDataTypeStr=boolean
  Mux3 : Mux  Inputs=2
  PLL (3ph)1 : Subsystem  DialogController=POWERSYS.PowerSysDialog  LoadFcn=sps_rtmsupport('LoadFcn', gcbh);  StartFcn=sps_rtmsupport('StartFcn', gcbh);  StopFcn=sps_rtmsupport('StopFcn', gcbh);  mask(PLL (3ph)){Flim=[55 66], Par_Init=[90, 60], ParK=[pll_kp, pll_ki, 1], TcD=Ts, MaxRateChangeFreq=12, FilterCutOffFreq=25, Ts=Ts, AGC=off}
      mask prompts: Flim "Minimum frequency (Hz):"; Par_Init "Initial inputs [ Phase (degrees), Frequency (Hz) ]:"; ParK "Regulator gains [ Kp, Ki, Kd ]:"; TcD "Time constant for derivative action (s):"; MaxRateChangeFreq "Maximum rate of change of frequency (Hz/s):"; FilterCutOffFreq "Filter cut-off frequency for frequency measurement (Hz):"; Ts "Sample time:"; AGC "Enable automatic gain control"
      mask help:
      | This Phase Locked Loop (PLL) system can be used  to synchronize on a set of variable frequency, three-phase sinusoidal signals. If the Automatic Gain Control is enabled, the input (phase error) of the PLL regulator is scaled according to the input signals magnitude.
      |
      | For optimal performance, set regulator gains [ Kp Ki  Kd ] = [ 180  3200  1 ] and check the Enable Automatic Gain Control parameter.
      |
      | Input : Vector containing the normalized three-phase signals [Va Vb Vc]
      | Output 1:  Measured frequency (Hz) = w/(2pi)
      | Output 2:  Ramp w.t varying between  0 and 2*pi, synchronized on zero crossings of the fundamental (positive-sequence) of phase A.
      mask init:
      | %block=gcb;
      | %[WantBlockChoice,Ts,sps] = powericon('PLL3phInit',block,Fmin,Par_Init,ParK,TcD, MaxRateChangeFreq, FilterCutOffFreq, AGC,Ts);
      | %powericon('SetInternalModels','set',block,WantBlockChoice);
      settings: CopyFcn=sps_rtmsupport('CopyFcn', gcbh);  DeleteFcn=sps_rtmsupport('DeleteFcn', gcbh);  UndoDeleteFcn=sps_rtmsupport('UndoDeleteFcn', gcbh);  ModelCloseFcn=sps_rtmsupport('ModelCloseFcn', gcbh);  PreSaveFcn=sps_rtmsupport('PreSaveFcn', gcbh);  PostSaveFcn=sps_rtmsupport('PostSaveFcn', gcbh);  NameChangeFcn=sps_rtmsupport('NameChangeFcn', gcbh);  PreCopyFcn=sps_rtmsupport('PreCopyFcn', gcbh);  CloseFcn=sps_rtmsupport('CloseFcn', gcbh);  PreDeleteFcn=sps_rtmsupport('PreDeleteFcn', gcbh);
      settings: OpenFcn=|
      | power_openblockproxy();
      | sps_rtmsupport('OpenFcn', gcbh, [8]);
      mask Help: helpview(psbhelp);
  Scope : Scope  NumInputPorts=5
  Selector1 : Selector  InputPortWidth=3  IndexOptions=Index vector (dialog)  Indices=1  OutputSizes=1
  Selector2 : Selector  InputPortWidth=3  IndexOptions=Index vector (dialog)  Indices=2  OutputSizes=1
  Selector3 : Selector  InputPortWidth=4  IndexOptions=Index vector (dialog)  Indices=[1]  OutputSizes=1
  Switch : Switch  Criteria=u2 > Threshold
  Terminator : Terminator
  Trigonometric Function2 : Trigonometry
  Trigonometric Function3 : Trigonometry  Operator=cos
  VCO : Subsystem
  tag scope: pll=scoped
  wires:
  Switch/1 -> Bus Creator/3, Scope/5, Trigonometric Function2/1, Trigonometric Function3/1  "wt"
  PLL (3ph)1/3(dq0) -> Selector2/1, Selector1/1
  Logical Operator7/1 -> Scope/1, [use_pll]  "use_pll"
  Logical Operator3/1 -> Logical Operator7/2
  Logical Operator5/1 -> Logical Operator3/2
  Logical Operator4/1 -> Logical Operator3/1
  Bus Selector10/1 -> Logical Operator5/1  "<GF_mode>"
  Logical Operator1/1 -> Logical Operator7/1
  [lock] -> Logical Operator1/2
  [cb_open] -> Logical Operator1/1, Scope/4, Logical Operator4/1  "cb_open"
  Bus Selector8/1 -> Logical Operator8/1  "<cb_status>"
  Logical Operator8/1 -> Display/1, [cb_open]
  [inputs] -> Bus Selector8/1
  [inputs] -> Bus Selector10/1
  Trigonometric Function3/1 -> Mux3/2
  Trigonometric Function2/1 -> Mux3/1
  Mux3/1 -> Bus Creator/4  "ejwt"
  Logical Operator6/1 -> Switch/2
  [use_pll] -> VCO/2(rst), Logical Operator6/1
  VCO/1(theta) -> Switch/1
  Gain1/1 -> VCO/1(w)
  [ref_lim] -> Selector3/1
  Selector3/1 -> Scope/3, Gain1/1
  Gain/1 -> Bus Creator/1  "freq"
  PLL (3ph)1/2(wt) -> VCO/3(init), Switch/3  "wt"
  Bus Selector2/1 -> PLL (3ph)1/1(abc)  "<vabc_line>"
  [cb_pu] -> Bus Selector2/1
  Data Type Conversion/1 -> DebounceAlternative/1(In)
  Constant/1 -> DebounceAlternative/2(Rst)
  DebounceAlternative/2(IntOut) -> Terminator/1
  Logical Operator2/1 -> Data Type Conversion/1
  Selector2/1 -> Aligned/1
  Selector1/1 -> Aligned1/1
  Aligned1/1 -> Logical Operator2/2
  Aligned/1 -> Logical Operator2/1
  DebounceAlternative/1(Out) -> Scope/2, [lock], Bus Creator/5  "lock"
  PLL (3ph)1/1(Freq) -> Gain/1, Bus Creator/2  "Freq"
  Bus Creator/1 -> [pll]

== system Microgrid_transition_model_111821_ben/FC_BESS/SMAInverter/85_SMAControl/InvControl/Ref_Limiting ==
  Constant : Constant
  Constant1 : Constant  Value=-1
  Demux : Demux
  RefLimiting : Subsystem
  Scope : Scope  NumInputPorts=4
  tag scope: ref_lim=scoped
  wires:
  Demux/4 -> Scope/4
  Demux/3 -> Scope/3
  Demux/2 -> Scope/2
  Demux/1 -> Scope/1
  [droop] -> RefLimiting/1(fvpq_in)
  Constant/1 -> RefLimiting/2(p_max)
  Constant1/1 -> RefLimiting/3(p_min)
  RefLimiting/1(fvpq_out) -> Demux/1, [ref_lim]  "FVPQ"
